simulink model "dronemodel"  (R2023a)
settings: Solver=VariableStepAuto  StartTime=0.0  StopTime=300  RelTol=1e-3
values from neighbouring files (symbols this model uses):
  Ax = 1    [dronevalues.m]
  Ay = 1    [dronevalues.m]
  Az = 1    [dronevalues.m]
  b = 3.59*10^-5    (= 3.59e-05)    [dronevalues.m]
  d = 0.1    [dronevalues.m]
  g = 9.81    [dronevalues.m]
  h = 5    [dronevalues.m]
  Ixx = 0.00963    [dronevalues.m]
  Iyy = 0.00963    [dronevalues.m]
  Izz = 0.019    [dronevalues.m]
  Jr = 0.04439    [dronevalues.m]
  l = 0.24    [dronevalues.m]
  m = 0.9928    [dronevalues.m]
undefined symbols (not defined in the file or in its folder): JSBSim, Rascal110
libraries: SignalEditorBlockLib x9, simulink_extras x7, slpidlib x4, aerolibfltsims x2
settings Model: Creator=ASUS  LastModifiedBy=ASUS

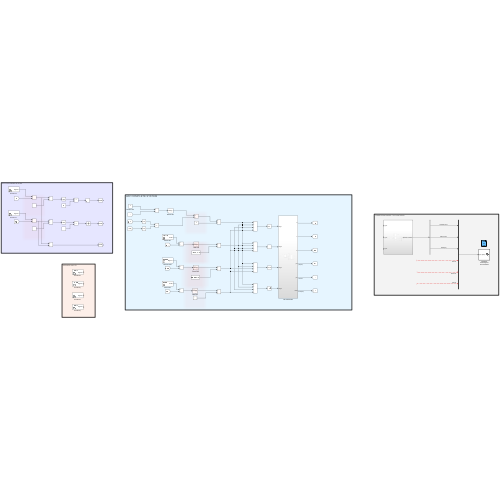
[thumbnail: Simulink's stored preview of the top-level diagram]
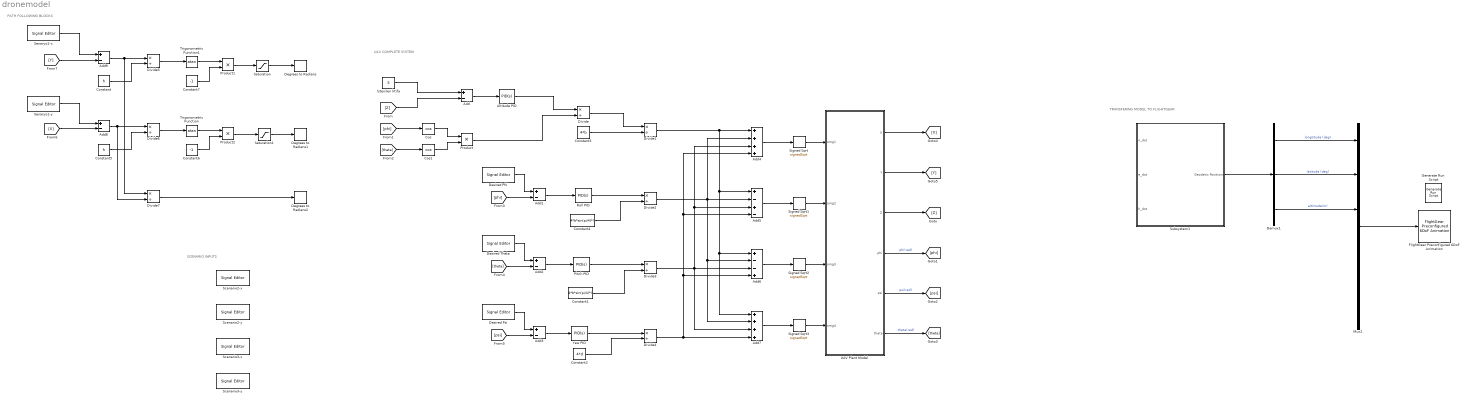
== system dronemodel ==
  note: UAV COMPLETE SYSTEM
  note: TRANSFERING MODEL TO FLIGHTGEAR
  note: PATH FOLLOWING BLOCKS
  note: SCENARIO INPUTS
  Add{,1..3,8..9} (6 alike) : Sum  Inputs=+-
  Add4 : Sum  Inputs=++++
  Add5 : Sum  Inputs=+-+-
  Add6 : Sum  Inputs=+--+
  Add7 : Sum  Inputs=++++
  Altitude PID : slpidlib/PID Controller  Controller=PID  Form=Parallel  TimeDomain=Continuous-time  UseExternalTs=off  SampleTime=-1  IntegratorMethod=Forward Euler  FilterMethod=Forward Euler  ControllerParametersSource=internal  P=1  I=1  UseKiTs=off  D=0  N=100  UseFilter=on  TunerSelectOption=Transfer Function Based (PID Tuner App)  InitialConditionSource=internal  InitialConditionForIntegrator=0  InitialConditionForFilter=0  DifferentiatorICPrevScaledInput=0  ExternalReset=none  TrackingMode=off  Kt=1  LimitOutput=off  SatLimitsSource=internal  UpperSaturationLimit=inf  LowerSaturationLimit=-inf  LinearizeAsGain=on  AntiWindupMode=none  Kb=1  LimitIntegrator=off  UpperIntegratorSaturationLimit=inf  LowerIntegratorSaturationLimit=-inf  POutMin=[]  POutMax=[]  IOutMin=[]  IOutMax=[]  DOutMin=[]  DOutMax=[]  NOutMin=[]  NOutMax=[]  SumOutMin=[]  SumOutMax=[]  SaturationOutMin=[]  SaturationOutMax=[]  PParamMin=[]  PParamMax=[]  IParamMin=[]  IParamMax=[]  DParamMin=[]  DParamMax=[]  NParamMin=[]  NParamMax=[]  KbParamMin=[]  KbParamMax=[]  KtParamMin=[]  KtParamMax=[]  KbOutMin=[]  KbOutMax=[]  KtOutMin=[]  KtOutMax=[]  IntegratorOutMin=[]  IntegratorOutMax=[]  FilterOutMin=[]  FilterOutMax=[]  SumI1OutMin=[]  SumI1OutMax=[]  SumI2OutMin=[]  SumI2OutMax=[]  SumI3OutMin=[]  SumI3OutMax=[]  SumI4OutMin=[]  SumI4OutMax=[]  SumDOutMin=[]  SumDOutMax=[]  DifferentiatorOutMin=[]  DifferentiatorOutMax=[]  FilterDiffOutCoefMin=[]  FilterDiffOutCoefMax=[]  ReciprocalOutMin=[]  ReciprocalOutMax=[]  SumDenOutMin=[]  SumDenOutMax=[]  SumNumOutMin=[]  SumNumOutMax=[]  DivideOutMin=[]  DivideOutMax=[]  UdiffTsProdOutMin=[]  UdiffTsProdOutMax=[]  NTsProdOutMin=[]  NTsProdOutMax=[]  UintegralTsProdOutMin=[]  UintegralTsProdOutMax=[]  UngainTsProdOutMin=[]  UngainTsProdOutMax=[]  ClampingZeroOutDataTypeStr=Inherit: Inherit via back propagation  ClampingZeroOutMin=[]  ClampingZeroOutMax=[]  FilterDenConstantOutDataTypeStr=Inherit: Inherit via back propagation  FilterDenConstantOutMin=[]  FilterDenConstantOutMax=[]  PCopyOutDataTypeStr=Inherit: Inherit via back propagation  PCopyOutMin=[]  PCopyOutMax=[]  NCopyOutDataTypeStr=Inherit: Inherit via back propagation  NCopyOutMin=[]  NCopyOutMax=[]  IntegratorContinuousStateAttributes=''  IntegratorStateMustResolveToSignalObject=off  IntegratorRTWStateStorageClass=Auto  FilterContinuousStateAttributes=''  FilterStateMustResolveToSignalObject=off  FilterRTWStateStorageClass=Auto  ParallelPVariant=InternalParameters  IdealPVariant=Disabled  IVariant=InternalParameters  DVariant=InternalParameters  IntegratorVariant=Continuous  SatVariant=Disabled  AWVariant=Passthrough  PCopyVariant=Disabled  TRVariant=Disabled  FdbkBlocksVariant=Forward  IdealPFdbkVariant=Disabled  SatFdbkVariant=Disabled  DerivativeFilterVariant=ContFilter  NVariant=InternalParameters  NCopyVariant=Disabled  FilterICVariant=InternalICsFilter  IntegratorICVariant=InternalICs  ExternalResetVariant=Disabled  TRSumVariant=Passthrough  SumFdbkVariant=Disabled  SumVariant=Sum_PID  TsampFilterVariant=InternalTs  TsampNgainVariant=Passthrough  TsampIntegralVariant=Disabled_SignalSpec  ExternalSaturationOutDataTypeStr=Inherit: Same as second input
  Constant : Constant  Value=h
  Constant1 : Constant  Value=4*b*sin(pi/4)*l
  Constant2 : Constant  Value=4*d
  Constant3 : Constant  Value=4*b
  Constant4 : Constant  Value=4*b*sin(pi/4)*l
  Constant5 : Constant  Value=h
  Constant6 : Constant  Value=-1
  Constant7 : Constant  Value=-1
  Cos : Trigonometry  Operator=cos
  Cos1 : Trigonometry  Operator=cos
  Degrees to Radians : simulink_extras/Transformations/Degrees to Radians
  Degrees to Radians1 : simulink_extras/Transformations/Degrees to Radians
  Degrees to Radians2 : simulink_extras/Transformations/Degrees to Radians
  Demux1 : Demux  Outputs=3
  Desired Phi : SignalEditorBlockLib/Signal Editor  FileName=phisignal.mat  ActiveScenario=Scenario  ActiveSignal=Pulse  IsBus=off  OutputBusObjectStr=Bus: BusObject  SampleTime=0  Interpolate=off  ZeroCross=off  OutputAfterFinalValue=Setting to zero  Unit=inherit  PreserveSignalName=on  ApplySigPropsToAllScenarios=on
  Desired Psi : SignalEditorBlockLib/Signal Editor  FileName=psisignal.mat  ActiveScenario=Scenario  ActiveSignal=Pulse  IsBus=off  OutputBusObjectStr=Bus: BusObject  SampleTime=0  Interpolate=off  ZeroCross=off  OutputAfterFinalValue=Setting to zero  Unit=inherit  PreserveSignalName=on  ApplySigPropsToAllScenarios=on
  Desired Theta : SignalEditorBlockLib/Signal Editor  FileName=untitled.mat  ActiveScenario=Scenario  ActiveSignal=Signal 1  IsBus=off  OutputBusObjectStr=Bus: BusObject  SampleTime=0  Interpolate=off  ZeroCross=off  OutputAfterFinalValue=Setting to zero  Unit=inherit  PreserveSignalName=on  ApplySigPropsToAllScenarios=on
  Divide{,1..7} (8 alike) : Product  Inputs=*/  RndMeth=Zero  SaturateOnIntegerOverflow=on
  FlightGear Preconfigured 6DoF Animation : aerolibfltsims/FlightGear Preconfigured 6DoF Animation  xFlightGearVersion=v2019.1  DestinationIpAddress=127.0.0.1  DestinationPort=5502  SampleTime=1/100  packetVersion=24
  Generate Run Script : aerolibfltsims/Generate Run Script  Architecture=Win64  dataFlow=Send  GeometryModelName=Rascal110-JSBSim  AirportId=LTAE  RunwayId=21  InitialAltitude=6000  InitialHeading=32  OffsetDistance=0  OffsetAzimuth=0  InstallScenery=on  DisableShaders=off  OriginAddress=127.0.0.1  DestinationPort=5502  OriginPort=5505  LocalAddress=127.0.0.1  OutputFileName=runfg.bat  FlightGearBaseDirectory=C:\FlightGear
  Mux2 : Mux  Inputs=6
  Pitch PID : slpidlib/PID Controller  Controller=PID  Form=Parallel  TimeDomain=Continuous-time  UseExternalTs=off  SampleTime=-1  IntegratorMethod=Forward Euler  FilterMethod=Forward Euler  ControllerParametersSource=internal  P=1  I=1  UseKiTs=off  D=0  N=100  UseFilter=on  TunerSelectOption=Transfer Function Based (PID Tuner App)  InitialConditionSource=internal  InitialConditionForIntegrator=0  InitialConditionForFilter=0  DifferentiatorICPrevScaledInput=0  ExternalReset=none  TrackingMode=off  Kt=1  LimitOutput=off  SatLimitsSource=internal  UpperSaturationLimit=inf  LowerSaturationLimit=-inf  LinearizeAsGain=on  AntiWindupMode=none  Kb=1  LimitIntegrator=off  UpperIntegratorSaturationLimit=inf  LowerIntegratorSaturationLimit=-inf  POutMin=[]  POutMax=[]  IOutMin=[]  IOutMax=[]  DOutMin=[]  DOutMax=[]  NOutMin=[]  NOutMax=[]  SumOutMin=[]  SumOutMax=[]  SaturationOutMin=[]  SaturationOutMax=[]  PParamMin=[]  PParamMax=[]  IParamMin=[]  IParamMax=[]  DParamMin=[]  DParamMax=[]  NParamMin=[]  NParamMax=[]  KbParamMin=[]  KbParamMax=[]  KtParamMin=[]  KtParamMax=[]  KbOutMin=[]  KbOutMax=[]  KtOutMin=[]  KtOutMax=[]  IntegratorOutMin=[]  IntegratorOutMax=[]  FilterOutMin=[]  FilterOutMax=[]  SumI1OutMin=[]  SumI1OutMax=[]  SumI2OutMin=[]  SumI2OutMax=[]  SumI3OutMin=[]  SumI3OutMax=[]  SumI4OutMin=[]  SumI4OutMax=[]  SumDOutMin=[]  SumDOutMax=[]  DifferentiatorOutMin=[]  DifferentiatorOutMax=[]  FilterDiffOutCoefMin=[]  FilterDiffOutCoefMax=[]  ReciprocalOutMin=[]  ReciprocalOutMax=[]  SumDenOutMin=[]  SumDenOutMax=[]  SumNumOutMin=[]  SumNumOutMax=[]  DivideOutMin=[]  DivideOutMax=[]  UdiffTsProdOutMin=[]  UdiffTsProdOutMax=[]  NTsProdOutMin=[]  NTsProdOutMax=[]  UintegralTsProdOutMin=[]  UintegralTsProdOutMax=[]  UngainTsProdOutMin=[]  UngainTsProdOutMax=[]  ClampingZeroOutDataTypeStr=Inherit: Inherit via back propagation  ClampingZeroOutMin=[]  ClampingZeroOutMax=[]  FilterDenConstantOutDataTypeStr=Inherit: Inherit via back propagation  FilterDenConstantOutMin=[]  FilterDenConstantOutMax=[]  PCopyOutDataTypeStr=Inherit: Inherit via back propagation  PCopyOutMin=[]  PCopyOutMax=[]  NCopyOutDataTypeStr=Inherit: Inherit via back propagation  NCopyOutMin=[]  NCopyOutMax=[]  IntegratorContinuousStateAttributes=''  IntegratorStateMustResolveToSignalObject=off  IntegratorRTWStateStorageClass=Auto  FilterContinuousStateAttributes=''  FilterStateMustResolveToSignalObject=off  FilterRTWStateStorageClass=Auto  ParallelPVariant=InternalParameters  IdealPVariant=Disabled  IVariant=InternalParameters  DVariant=InternalParameters  IntegratorVariant=Continuous  SatVariant=Disabled  AWVariant=Passthrough  PCopyVariant=Disabled  TRVariant=Disabled  FdbkBlocksVariant=Forward  IdealPFdbkVariant=Disabled  SatFdbkVariant=Disabled  DerivativeFilterVariant=ContFilter  NVariant=InternalParameters  NCopyVariant=Disabled  FilterICVariant=InternalICsFilter  IntegratorICVariant=InternalICs  ExternalResetVariant=Disabled  TRSumVariant=Passthrough  SumFdbkVariant=Disabled  SumVariant=Sum_PID  TsampFilterVariant=InternalTs  TsampNgainVariant=Passthrough  TsampIntegralVariant=Disabled_SignalSpec  ExternalSaturationOutDataTypeStr=Inherit: Same as second input
  Product : Product
  Product1 : Product
  Product2 : Product
  Roll PID : slpidlib/PID Controller  Controller=PID  Form=Parallel  TimeDomain=Continuous-time  UseExternalTs=off  SampleTime=-1  IntegratorMethod=Forward Euler  FilterMethod=Forward Euler  ControllerParametersSource=internal  P=1  I=1  UseKiTs=off  D=0  N=100  UseFilter=on  TunerSelectOption=Transfer Function Based (PID Tuner App)  InitialConditionSource=internal  InitialConditionForIntegrator=0  InitialConditionForFilter=0  DifferentiatorICPrevScaledInput=0  ExternalReset=none  TrackingMode=off  Kt=1  LimitOutput=off  SatLimitsSource=internal  UpperSaturationLimit=inf  LowerSaturationLimit=-inf  LinearizeAsGain=on  AntiWindupMode=none  Kb=1  LimitIntegrator=off  UpperIntegratorSaturationLimit=inf  LowerIntegratorSaturationLimit=-inf  POutMin=[]  POutMax=[]  IOutMin=[]  IOutMax=[]  DOutMin=[]  DOutMax=[]  NOutMin=[]  NOutMax=[]  SumOutMin=[]  SumOutMax=[]  SaturationOutMin=[]  SaturationOutMax=[]  PParamMin=[]  PParamMax=[]  IParamMin=[]  IParamMax=[]  DParamMin=[]  DParamMax=[]  NParamMin=[]  NParamMax=[]  KbParamMin=[]  KbParamMax=[]  KtParamMin=[]  KtParamMax=[]  KbOutMin=[]  KbOutMax=[]  KtOutMin=[]  KtOutMax=[]  IntegratorOutMin=[]  IntegratorOutMax=[]  FilterOutMin=[]  FilterOutMax=[]  SumI1OutMin=[]  SumI1OutMax=[]  SumI2OutMin=[]  SumI2OutMax=[]  SumI3OutMin=[]  SumI3OutMax=[]  SumI4OutMin=[]  SumI4OutMax=[]  SumDOutMin=[]  SumDOutMax=[]  DifferentiatorOutMin=[]  DifferentiatorOutMax=[]  FilterDiffOutCoefMin=[]  FilterDiffOutCoefMax=[]  ReciprocalOutMin=[]  ReciprocalOutMax=[]  SumDenOutMin=[]  SumDenOutMax=[]  SumNumOutMin=[]  SumNumOutMax=[]  DivideOutMin=[]  DivideOutMax=[]  UdiffTsProdOutMin=[]  UdiffTsProdOutMax=[]  NTsProdOutMin=[]  NTsProdOutMax=[]  UintegralTsProdOutMin=[]  UintegralTsProdOutMax=[]  UngainTsProdOutMin=[]  UngainTsProdOutMax=[]  ClampingZeroOutDataTypeStr=Inherit: Inherit via back propagation  ClampingZeroOutMin=[]  ClampingZeroOutMax=[]  FilterDenConstantOutDataTypeStr=Inherit: Inherit via back propagation  FilterDenConstantOutMin=[]  FilterDenConstantOutMax=[]  PCopyOutDataTypeStr=Inherit: Inherit via back propagation  PCopyOutMin=[]  PCopyOutMax=[]  NCopyOutDataTypeStr=Inherit: Inherit via back propagation  NCopyOutMin=[]  NCopyOutMax=[]  IntegratorContinuousStateAttributes=''  IntegratorStateMustResolveToSignalObject=off  IntegratorRTWStateStorageClass=Auto  FilterContinuousStateAttributes=''  FilterStateMustResolveToSignalObject=off  FilterRTWStateStorageClass=Auto  ParallelPVariant=InternalParameters  IdealPVariant=Disabled  IVariant=InternalParameters  DVariant=InternalParameters  IntegratorVariant=Continuous  SatVariant=Disabled  AWVariant=Passthrough  PCopyVariant=Disabled  TRVariant=Disabled  FdbkBlocksVariant=Forward  IdealPFdbkVariant=Disabled  SatFdbkVariant=Disabled  DerivativeFilterVariant=ContFilter  NVariant=InternalParameters  NCopyVariant=Disabled  FilterICVariant=InternalICsFilter  IntegratorICVariant=InternalICs  ExternalResetVariant=Disabled  TRSumVariant=Passthrough  SumFdbkVariant=Disabled  SumVariant=Sum_PID  TsampFilterVariant=InternalTs  TsampNgainVariant=Passthrough  TsampIntegralVariant=Disabled_SignalSpec  ExternalSaturationOutDataTypeStr=Inherit: Same as second input
  Saturation : Saturate  UpperLimit=20  LowerLimit=-20
  Saturation1 : Saturate  UpperLimit=20  LowerLimit=-20
  Scenario2-x : SignalEditorBlockLib/Signal Editor  FileName=Senaryo2X.mat  ActiveScenario=Scenario  ActiveSignal=Signal 1  IsBus=off  OutputBusObjectStr=Bus: BusObject  SampleTime=0  Interpolate=off  ZeroCross=off  OutputAfterFinalValue=Setting to zero  Unit=inherit  PreserveSignalName=on  ApplySigPropsToAllScenarios=on
  Scenario2-y : SignalEditorBlockLib/Signal Editor  FileName=C:\Users\s22734\Desktop\Senaryo2Y.mat  ActiveScenario=Scenario  ActiveSignal=Signal 1  IsBus=off  OutputBusObjectStr=Bus: BusObject  SampleTime=0  Interpolate=off  ZeroCross=off  OutputAfterFinalValue=Setting to zero  Unit=inherit  PreserveSignalName=on  ApplySigPropsToAllScenarios=on
  Scenario3-x : SignalEditorBlockLib/Signal Editor  FileName=Senaryo3X.mat  ActiveScenario=Scenario  ActiveSignal=Signal 1  IsBus=off  OutputBusObjectStr=Bus: BusObject  SampleTime=0  Interpolate=off  ZeroCross=off  OutputAfterFinalValue=Setting to zero  Unit=inherit  PreserveSignalName=on  ApplySigPropsToAllScenarios=on
  Scenario3-y : SignalEditorBlockLib/Signal Editor  FileName=Senaryo3Y.mat  ActiveScenario=Scenario  ActiveSignal=Signal 1  IsBus=off  OutputBusObjectStr=Bus: BusObject  SampleTime=0  Interpolate=off  ZeroCross=off  OutputAfterFinalValue=Setting to zero  Unit=inherit  PreserveSignalName=on  ApplySigPropsToAllScenarios=on
  Senaryo1-x : SignalEditorBlockLib/Signal Editor  FileName=C:\Users\s22734\Desktop\Senaryo1X.mat  ActiveScenario=Scenario  ActiveSignal=Signal 1  IsBus=off  OutputBusObjectStr=Bus: BusObject  SampleTime=0  Interpolate=off  ZeroCross=off  OutputAfterFinalValue=Setting to zero  Unit=inherit  PreserveSignalName=on  ApplySigPropsToAllScenarios=on
  Senaryo1-y : SignalEditorBlockLib/Signal Editor  FileName=C:\Users\s22734\Desktop\Senaryo1Y.mat  ActiveScenario=Scenario  ActiveSignal=Signal 1  IsBus=off  OutputBusObjectStr=Bus: BusObject  SampleTime=0  Interpolate=off  ZeroCross=off  OutputAfterFinalValue=Setting to zero  Unit=inherit  PreserveSignalName=on  ApplySigPropsToAllScenarios=on
  Signed Sqrt{,1..3} (4 alike) : Sqrt  Operator=signedSqrt
  Subsystem1 : Subsystem
  Trigonometric Function : Trigonometry  Operator=atan
  Trigonometric Function1 : Trigonometry  Operator=atan
  UAV Plant Model : Subsystem
  Yaw PID : slpidlib/PID Controller  Controller=PID  Form=Parallel  TimeDomain=Continuous-time  UseExternalTs=off  SampleTime=-1  IntegratorMethod=Forward Euler  FilterMethod=Forward Euler  ControllerParametersSource=internal  P=1  I=1  UseKiTs=off  D=0  N=100  UseFilter=on  TunerSelectOption=Transfer Function Based (PID Tuner App)  InitialConditionSource=internal  InitialConditionForIntegrator=0  InitialConditionForFilter=0  DifferentiatorICPrevScaledInput=0  ExternalReset=none  TrackingMode=off  Kt=1  LimitOutput=off  SatLimitsSource=internal  UpperSaturationLimit=inf  LowerSaturationLimit=-inf  LinearizeAsGain=on  AntiWindupMode=none  Kb=1  LimitIntegrator=off  UpperIntegratorSaturationLimit=inf  LowerIntegratorSaturationLimit=-inf  POutMin=[]  POutMax=[]  IOutMin=[]  IOutMax=[]  DOutMin=[]  DOutMax=[]  NOutMin=[]  NOutMax=[]  SumOutMin=[]  SumOutMax=[]  SaturationOutMin=[]  SaturationOutMax=[]  PParamMin=[]  PParamMax=[]  IParamMin=[]  IParamMax=[]  DParamMin=[]  DParamMax=[]  NParamMin=[]  NParamMax=[]  KbParamMin=[]  KbParamMax=[]  KtParamMin=[]  KtParamMax=[]  KbOutMin=[]  KbOutMax=[]  KtOutMin=[]  KtOutMax=[]  IntegratorOutMin=[]  IntegratorOutMax=[]  FilterOutMin=[]  FilterOutMax=[]  SumI1OutMin=[]  SumI1OutMax=[]  SumI2OutMin=[]  SumI2OutMax=[]  SumI3OutMin=[]  SumI3OutMax=[]  SumI4OutMin=[]  SumI4OutMax=[]  SumDOutMin=[]  SumDOutMax=[]  DifferentiatorOutMin=[]  DifferentiatorOutMax=[]  FilterDiffOutCoefMin=[]  FilterDiffOutCoefMax=[]  ReciprocalOutMin=[]  ReciprocalOutMax=[]  SumDenOutMin=[]  SumDenOutMax=[]  SumNumOutMin=[]  SumNumOutMax=[]  DivideOutMin=[]  DivideOutMax=[]  UdiffTsProdOutMin=[]  UdiffTsProdOutMax=[]  NTsProdOutMin=[]  NTsProdOutMax=[]  UintegralTsProdOutMin=[]  UintegralTsProdOutMax=[]  UngainTsProdOutMin=[]  UngainTsProdOutMax=[]  ClampingZeroOutDataTypeStr=Inherit: Inherit via back propagation  ClampingZeroOutMin=[]  ClampingZeroOutMax=[]  FilterDenConstantOutDataTypeStr=Inherit: Inherit via back propagation  FilterDenConstantOutMin=[]  FilterDenConstantOutMax=[]  PCopyOutDataTypeStr=Inherit: Inherit via back propagation  PCopyOutMin=[]  PCopyOutMax=[]  NCopyOutDataTypeStr=Inherit: Inherit via back propagation  NCopyOutMin=[]  NCopyOutMax=[]  IntegratorContinuousStateAttributes=''  IntegratorStateMustResolveToSignalObject=off  IntegratorRTWStateStorageClass=Auto  FilterContinuousStateAttributes=''  FilterStateMustResolveToSignalObject=off  FilterRTWStateStorageClass=Auto  ParallelPVariant=InternalParameters  IdealPVariant=Disabled  IVariant=InternalParameters  DVariant=InternalParameters  IntegratorVariant=Continuous  SatVariant=Disabled  AWVariant=Passthrough  PCopyVariant=Disabled  TRVariant=Disabled  FdbkBlocksVariant=Forward  IdealPFdbkVariant=Disabled  SatFdbkVariant=Disabled  DerivativeFilterVariant=ContFilter  NVariant=InternalParameters  NCopyVariant=Disabled  FilterICVariant=InternalICsFilter  IntegratorICVariant=InternalICs  ExternalResetVariant=Disabled  TRSumVariant=Passthrough  SumFdbkVariant=Disabled  SumVariant=Sum_PID  TsampFilterVariant=InternalTs  TsampNgainVariant=Passthrough  TsampIntegralVariant=Disabled_SignalSpec  ExternalSaturationOutDataTypeStr=Inherit: Same as second input
  İstenilen İrtifa : Constant  Value=5
  wires:
  Add4/1 -> Signed Sqrt/1
  Add5/1 -> Signed Sqrt1/1
  Add6/1 -> Signed Sqrt2/1
  Add7/1 -> Signed Sqrt3/1
  UAV Plant Model/1(X) -> [X]
  UAV Plant Model/2(Y) -> [Y]
  İstenilen İrtifa/1 -> Add/1
  Add/1 -> Altitude PID/1
  UAV Plant Model/3(Z) -> [Z]
  [Z] -> Add/2
  [phi] -> Cos/1
  [theta] -> Cos1/1
  Cos/1 -> Product/1
  Cos1/1 -> Product/2
  Product/1 -> Divide/2
  Altitude PID/1 -> Divide/1
  [phi] -> Add1/2
  Add1/1 -> Roll PID/1
  [theta] -> Add2/2
  Add2/1 -> Pitch PID/1
  [psi] -> Add3/2
  Add3/1 -> Yaw PID/1
  Divide/1 -> Divide1/1
  Constant3/1 -> Divide1/2
  Roll PID/1 -> Divide2/1
  Constant4/1 -> Divide2/2
  Pitch PID/1 -> Divide3/1
  Constant1/1 -> Divide3/2
  Yaw PID/1 -> Divide4/1
  Constant2/1 -> Divide4/2
  Divide1/1 -> Add6/1, Add7/1, Add5/1, Add4/1
  Divide2/1 -> Add7/2, Add6/2, Add5/2, Add4/2
  Divide4/1 -> Add4/4, Add5/4, Add6/4, Add7/4
  Divide3/1 -> Add7/3, Add6/3, Add4/3, Add5/3
  Signed Sqrt/1 -> UAV Plant Model/1(omg1)
  Signed Sqrt1/1 -> UAV Plant Model/2(omg2)
  Signed Sqrt2/1 -> UAV Plant Model/3(omg3)
  Signed Sqrt3/1 -> UAV Plant Model/4(omg4)
  ? -> Mux2/5  "theta(rad)"
  Demux1/2 -> Mux2/2  "latitude (deg)"
  Demux1/1 -> Mux2/1  "longtitude (deg)"
  Mux2/1 -> FlightGear Preconfigured 6DoF Animation/1
  ? -> Mux2/6  "psi(rad)"
  ? -> Mux2/4  "phi(rad)"
  Demux1/3 -> Mux2/3  "altittude(m)"
  Subsystem1/1(Geodetic Positions) -> Demux1/1
  [X] -> Add8/2
  [Y] -> Add9/2
  Add9/1 -> Divide5/1, Divide7/1
  Add8/1 -> Divide6/1, Divide7/2
  Constant/1 -> Divide5/2
  Constant5/1 -> Divide6/2
  Divide5/1 -> Trigonometric Function1/1
  Divide6/1 -> Trigonometric Function/1
  Trigonometric Function1/1 -> Product1/1
  Trigonometric Function/1 -> Product2/1
  Senaryo1-x/1 -> Add9/1
  Senaryo1-y/1 -> Add8/1
  Product1/1 -> Saturation/1
  Product2/1 -> Saturation1/1
  Constant7/1 -> Product1/2
  Constant6/1 -> Product2/2
  Saturation/1 -> Degrees to Radians/1
  Saturation1/1 -> Degrees to Radians1/1
  Divide7/1 -> Degrees to Radians2/1
  UAV Plant Model/4(phi) -> [phi]  "phi(rad)"
  UAV Plant Model/5(psi) -> [psi]  "psi(rad)"
  UAV Plant Model/6(theta) -> [theta]  "theta(rad)"
  Desired Phi/1 -> Add1/1
  Desired Theta/1 -> Add2/1
  Desired Psi/1 -> Add3/1

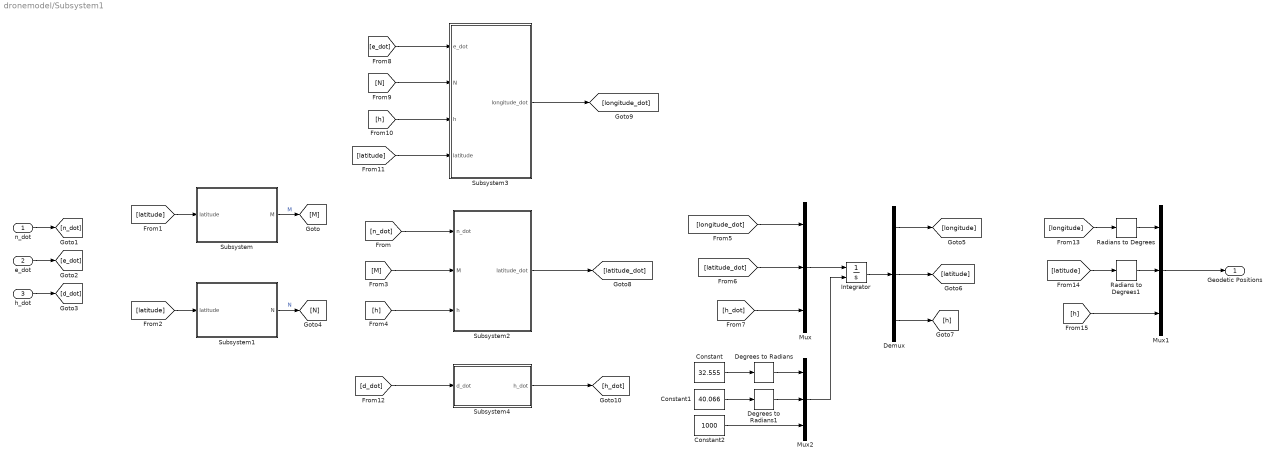
== system dronemodel/Subsystem1 ==
  n_dot : Inport
  e_dot : Inport  Port=2
  h_dot : Inport  Port=3
  Constant : Constant  Value=32.555
  Constant1 : Constant  Value=40.066
  Constant2 : Constant  Value=1000
  Degrees to Radians : simulink_extras/Transformations/Degrees to Radians
  Degrees to Radians1 : simulink_extras/Transformations/Degrees to Radians
  Demux : Demux  Outputs=3
  Integrator : Integrator  InitialConditionSource=external  InitialCondition=[32.555;40.066;3000]
  Mux : Mux  Inputs=3
  Mux1 : Mux  Inputs=3
  Mux2 : Mux  Inputs=3
  Radians to Degrees : simulink_extras/Transformations/Radians to Degrees
  Radians to Degrees1 : simulink_extras/Transformations/Radians to Degrees
  Subsystem : Subsystem
  Subsystem1 : Subsystem
  Subsystem2 : Subsystem
  Subsystem3 : Subsystem
  Subsystem4 : Subsystem
  Geodetic Positions : Outport
  wires:
  e_dot/1 -> [e_dot]
  n_dot/1 -> [n_dot]
  h_dot/1 -> [d_dot]
  [latitude] -> Subsystem/1(latitude)
  Subsystem/1(M) -> [M]  "M"
  [latitude] -> Subsystem1/1(latitude)
  Subsystem1/1(N) -> [N]  "N"
  [longitude_dot] -> Mux/1
  [latitude_dot] -> Mux/2
  [h_dot] -> Mux/3
  Mux/1 -> Integrator/1
  Integrator/1 -> Demux/1
  Demux/1 -> [longitude]
  Demux/3 -> [h]
  Demux/2 -> [latitude]
  [n_dot] -> Subsystem2/1(n_dot)
  [M] -> Subsystem2/2(M)
  [h] -> Subsystem2/3(h)
  Subsystem2/1(latitude_dot) -> [latitude_dot]
  [e_dot] -> Subsystem3/1(e_dot)
  [N] -> Subsystem3/2(N)
  [h] -> Subsystem3/3(h)
  [latitude] -> Subsystem3/4(latitude)
  Subsystem3/1(longitude_dot) -> [longitude_dot]
  [d_dot] -> Subsystem4/1(d_dot)
  Subsystem4/1(h_dot) -> [h_dot]
  Mux1/1 -> Geodetic Positions/1
  [longitude] -> Radians to Degrees/1
  [latitude] -> Radians to Degrees1/1
  [h] -> Mux1/3
  Radians to Degrees1/1 -> Mux1/2
  Radians to Degrees/1 -> Mux1/1
  Constant/1 -> Degrees to Radians/1
  Degrees to Radians/1 -> Mux2/1
  Constant1/1 -> Degrees to Radians1/1
  Degrees to Radians1/1 -> Mux2/2
  Constant2/1 -> Mux2/3
  Mux2/1 -> Integrator/2

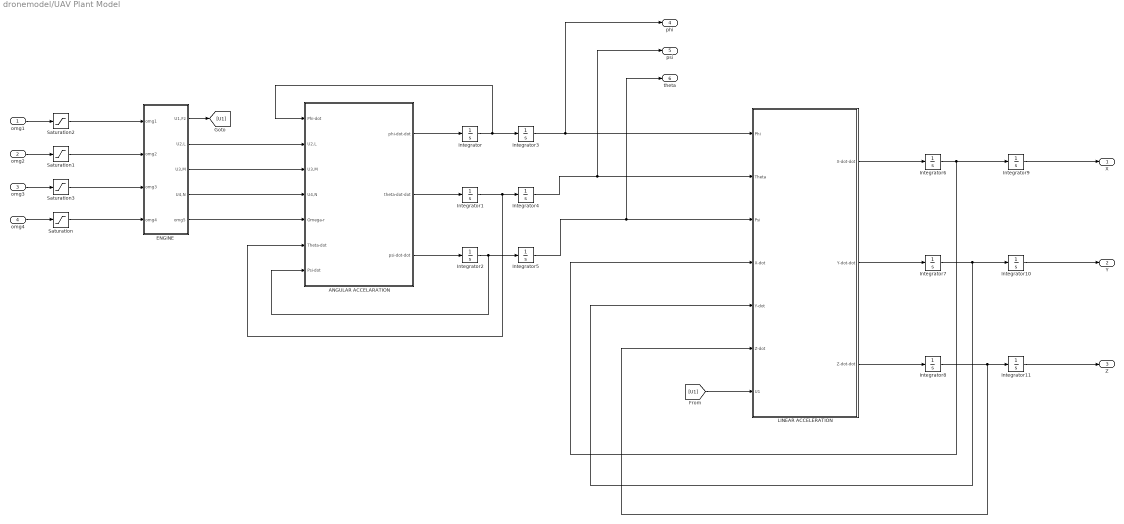
== system dronemodel/UAV Plant Model ==
  omg1 : Inport
  omg2 : Inport  Port=2
  omg3 : Inport  Port=3
  omg4 : Inport  Port=4
  ANGULAR ACCELARATION : Subsystem
  ENGINE : Subsystem
  Integrator{,1..2,6..10} (8 alike) : Integrator
  Integrator11 : Integrator  LimitOutput=on  LowerSaturationLimit=0
  Integrator3 : Integrator  WrapState=on
  Integrator4 : Integrator  WrapState=on
  Integrator5 : Integrator  WrapState=on
  LINEAR ACCELERATION : Subsystem
  Saturation{,1..3} (4 alike) : Saturate
  X : Outport
  Y : Outport  Port=2
  Z : Outport  Port=3
  phi : Outport  Port=4
  psi : Outport  Port=5
  theta : Outport  Port=6
  wires:
  ENGINE/4(U4,N) -> ANGULAR ACCELARATION/4(U4,N)
  Integrator11/1 -> Z/1
  Integrator2/1 -> ANGULAR ACCELARATION/7(Psi-dot), Integrator5/1
  Integrator1/1 -> ANGULAR ACCELARATION/6(Theta-dot), Integrator4/1
  Integrator7/1 -> LINEAR ACCELERATION/5(Y-dot), Integrator10/1
  ENGINE/2(U2,L) -> ANGULAR ACCELARATION/2(U2,L)
  omg1/1 -> Saturation2/1
  Integrator5/1 -> theta/1, LINEAR ACCELERATION/3(Psi)
  LINEAR ACCELERATION/3(Z-dot-dot) -> Integrator8/1
  omg3/1 -> Saturation3/1
  ENGINE/3(U3,M) -> ANGULAR ACCELARATION/3(U3,M)
  omg2/1 -> Saturation1/1
  Integrator/1 -> ANGULAR ACCELARATION/1(Phi-dot), Integrator3/1
  ENGINE/1(U1,Fz) -> [U1]
  Integrator10/1 -> Y/1
  Integrator6/1 -> LINEAR ACCELERATION/4(X-dot), Integrator9/1
  ENGINE/5(omg5) -> ANGULAR ACCELARATION/5(Omega-r)
  [U1] -> LINEAR ACCELERATION/7(U1)
  ANGULAR ACCELARATION/1(phi-dot-dot) -> Integrator/1
  ANGULAR ACCELARATION/3(psi-dot-dot) -> Integrator2/1
  Integrator4/1 -> psi/1, LINEAR ACCELERATION/2(Theta)
  Integrator9/1 -> X/1
  LINEAR ACCELERATION/2(Y-dot-dot) -> Integrator7/1
  Integrator3/1 -> phi/1, LINEAR ACCELERATION/1(Phi)
  omg4/1 -> Saturation/1
  ANGULAR ACCELARATION/2(theta-dot-dot) -> Integrator1/1
  LINEAR ACCELERATION/1(X-dot-dot) -> Integrator6/1
  Integrator8/1 -> LINEAR ACCELERATION/6(Z-dot), Integrator11/1
  Saturation1/1 -> ENGINE/2(omg2)
  Saturation2/1 -> ENGINE/1(omg1)
  Saturation3/1 -> ENGINE/3(omg3)
  Saturation/1 -> ENGINE/4(omg4)

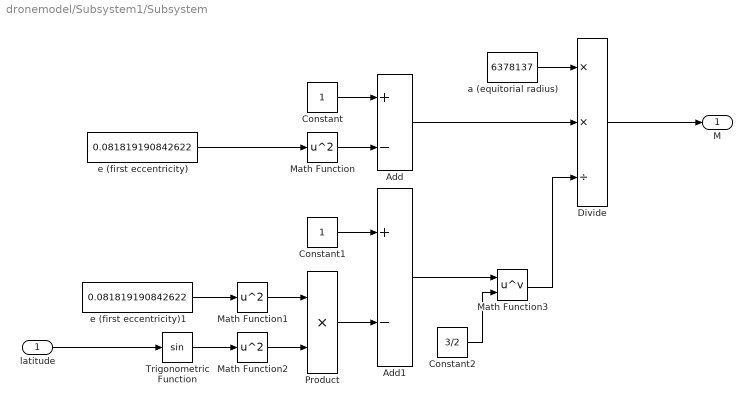
== system dronemodel/Subsystem1/Subsystem ==
  latitude : Inport
  Add : Sum  Inputs=+-
  Add1 : Sum  Inputs=+-
  Constant : Constant
  Constant1 : Constant
  Constant2 : Constant  Value=3/2
  Divide : Product  Inputs=**/
  Math Function : Math  Operator=square
  Math Function1 : Math  Operator=square
  Math Function2 : Math  Operator=square
  Math Function3 : Math  Operator=pow
  Product : Product
  Trigonometric Function : Trigonometry
  a (equitorial radius) : Constant  Value=6378137
  e (first eccentricity) : Constant  Value=0.081819190842622
  e (first eccentricity)1 : Constant  Value=0.081819190842622
  M : Outport
  wires:
  Constant1/1 -> Add1/1
  Add/1 -> Divide/2
  Add1/1 -> Math Function3/1
  Constant2/1 -> Math Function3/2
  Product/1 -> Add1/2
  a (equitorial radius)/1 -> Divide/1
  e (first eccentricity)1/1 -> Math Function1/1
  latitude/1 -> Trigonometric Function/1
  Math Function/1 -> Add/2
  Constant/1 -> Add/1
  Trigonometric Function/1 -> Math Function2/1
  e (first eccentricity)/1 -> Math Function/1
  Math Function1/1 -> Product/1
  Math Function2/1 -> Product/2
  Math Function3/1 -> Divide/3
  Divide/1 -> M/1

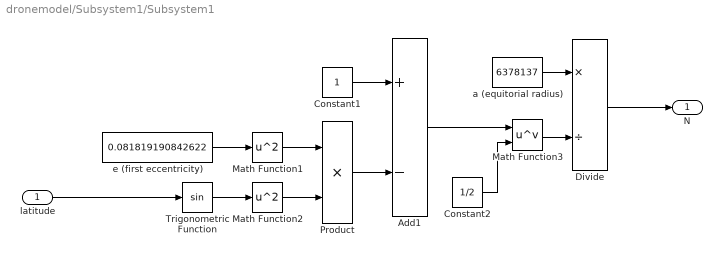
== system dronemodel/Subsystem1/Subsystem1 ==
  latitude : Inport
  Add1 : Sum  Inputs=+-
  Constant1 : Constant
  Constant2 : Constant  Value=1/2
  Divide : Product  Inputs=*/
  Math Function1 : Math  Operator=square
  Math Function2 : Math  Operator=square
  Math Function3 : Math  Operator=pow
  Product : Product
  Trigonometric Function : Trigonometry
  a (equitorial radius) : Constant  Value=6378137
  e (first eccentricity) : Constant  Value=0.081819190842622
  N : Outport
  wires:
  Math Function1/1 -> Product/1
  Product/1 -> Add1/2
  Constant2/1 -> Math Function3/2
  Constant1/1 -> Add1/1
  Add1/1 -> Math Function3/1
  latitude/1 -> Trigonometric Function/1
  Math Function3/1 -> Divide/2
  Math Function2/1 -> Product/2
  Trigonometric Function/1 -> Math Function2/1
  e (first eccentricity)/1 -> Math Function1/1
  a (equitorial radius)/1 -> Divide/1
  Divide/1 -> N/1

== system dronemodel/Subsystem1/Subsystem2 ==
  n_dot : Inport
  M : Inport  Port=2
  h : Inport  Port=3
  Add : Sum
  Divide : Product  Inputs=*/
  latitude_dot : Outport
  wires:
  Add/1 -> Divide/2
  Divide/1 -> latitude_dot/1
  M/1 -> Add/1
  n_dot/1 -> Divide/1
  h/1 -> Add/2

== system dronemodel/Subsystem1/Subsystem3 ==
  e_dot : Inport
  N : Inport  Port=2
  h : Inport  Port=3
  latitude : Inport  Port=4
  Add : Sum
  Divide : Product  Inputs=*//
  Trigonometric Function : Trigonometry  Operator=cos
  longitude_dot : Outport
  wires:
  Trigonometric Function/1 -> Divide/3
  Divide/1 -> longitude_dot/1
  Add/1 -> Divide/2
  latitude/1 -> Trigonometric Function/1
  N/1 -> Add/1
  e_dot/1 -> Divide/1
  h/1 -> Add/2

== system dronemodel/Subsystem1/Subsystem4 ==
  d_dot : Inport
  Gain : Gain  Gain=-1
  h_dot : Outport
  wires:
  Gain/1 -> h_dot/1
  d_dot/1 -> Gain/1

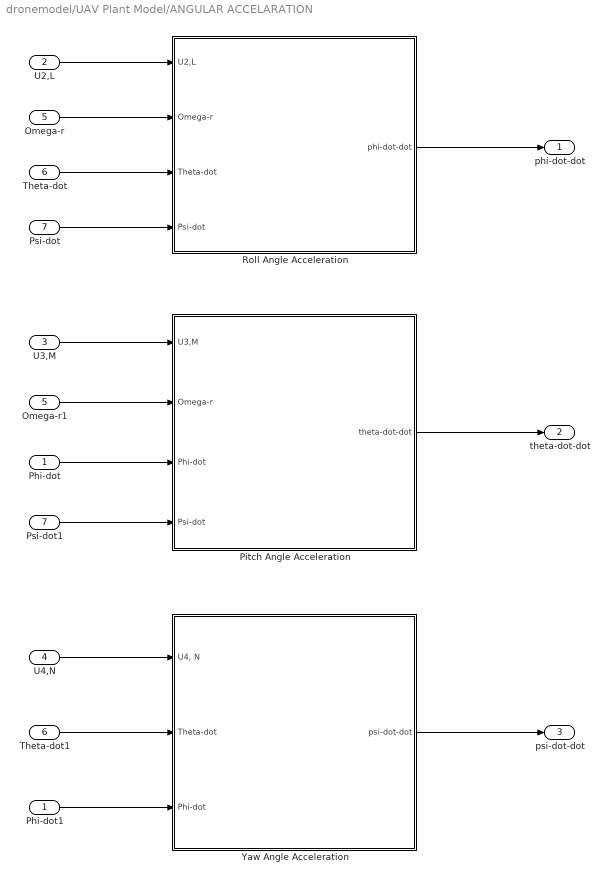
== system dronemodel/UAV Plant Model/ANGULAR ACCELARATION ==
  Phi-dot : Inport
  U2,L : Inport  Port=2
  U3,M : Inport  Port=3
  U4,N : Inport  Port=4
  Omega-r : Inport  Port=5
  Theta-dot : Inport  Port=6
  Psi-dot : Inport  Port=7
  Omega-r1 : InportShadow  Port=5
  Phi-dot1 : InportShadow
  Pitch Angle Acceleration : Subsystem
  Psi-dot1 : InportShadow  Port=7
  Roll Angle Acceleration : Subsystem
  Theta-dot1 : InportShadow  Port=6
  Yaw Angle Acceleration : Subsystem
  phi-dot-dot : Outport
  theta-dot-dot : Outport  Port=2
  psi-dot-dot : Outport  Port=3
  wires:
  U2,L/1 -> Roll Angle Acceleration/1(U2,L)
  Omega-r/1 -> Roll Angle Acceleration/2(Omega-r)
  Theta-dot/1 -> Roll Angle Acceleration/3(Theta-dot)
  Psi-dot/1 -> Roll Angle Acceleration/4(Psi-dot)
  Roll Angle Acceleration/1(phi-dot-dot) -> phi-dot-dot/1
  Pitch Angle Acceleration/1(theta-dot-dot) -> theta-dot-dot/1
  Yaw Angle Acceleration/1(psi-dot-dot) -> psi-dot-dot/1
  U3,M/1 -> Pitch Angle Acceleration/1(U3,M)
  Omega-r1/1 -> Pitch Angle Acceleration/2(Omega-r)
  Phi-dot/1 -> Pitch Angle Acceleration/3(Phi-dot)
  Psi-dot1/1 -> Pitch Angle Acceleration/4(Psi-dot)
  U4,N/1 -> Yaw Angle Acceleration/1("U4, N")
  Theta-dot1/1 -> Yaw Angle Acceleration/2(Theta-dot)
  Phi-dot1/1 -> Yaw Angle Acceleration/3(Phi-dot)

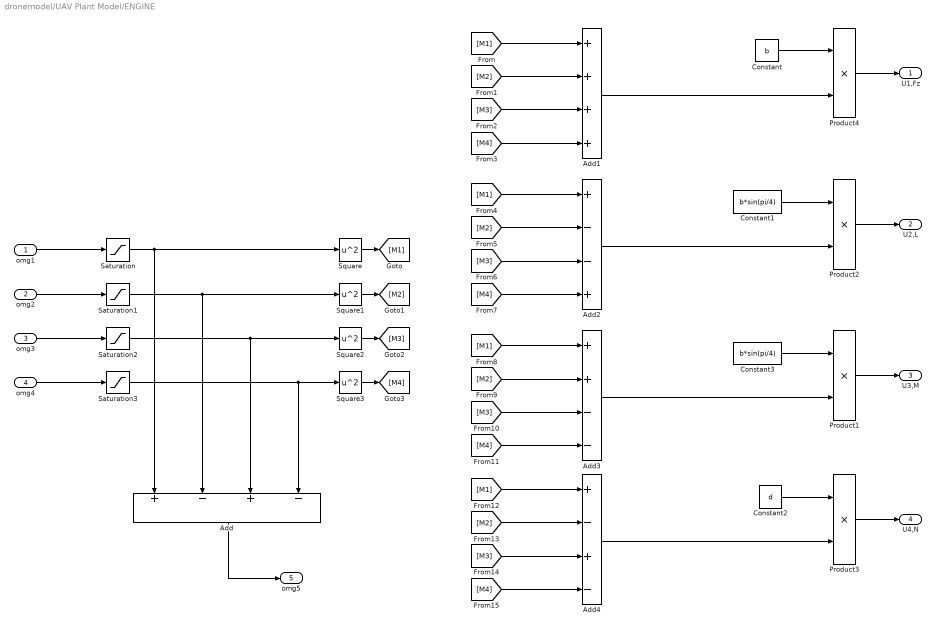
== system dronemodel/UAV Plant Model/ENGINE ==
  omg1 : Inport
  omg2 : Inport  Port=2
  omg3 : Inport  Port=3
  omg4 : Inport  Port=4
  Add : Sum  Inputs=+-+-
  Add1 : Sum  Inputs=++++
  Add2 : Sum  Inputs=+--+
  Add3 : Sum  Inputs=++--
  Add4 : Sum  Inputs=+-+-
  Constant : Constant  Value=b
  Constant1 : Constant  Value=b*sin(pi/4)
  Constant2 : Constant  Value=d
  Constant3 : Constant  Value=b*sin(pi/4)
  Product{1..4} (4 alike) : Product
  Saturation{,1..3} (4 alike) : Saturate
  Square{,1..3} (4 alike) : Math  Operator=square
  U1,Fz : Outport
  U2,L : Outport  Port=2
  U3,M : Outport  Port=3
  U4,N : Outport  Port=4
  omg5 : Outport  Port=5
  wires:
  omg1/1 -> Saturation/1
  omg3/1 -> Saturation2/1
  Saturation/1 -> Add/1, Square/1
  Saturation2/1 -> Add/3, Square2/1
  Saturation3/1 -> Add/4, Square3/1
  omg4/1 -> Saturation3/1
  Square1/1 -> [M2]
  Saturation1/1 -> Add/2, Square1/1
  Square2/1 -> [M3]
  Square/1 -> [M1]
  Square3/1 -> [M4]
  omg2/1 -> Saturation1/1
  Add/1 -> omg5/1
  [M1] -> Add1/1
  [M2] -> Add1/2
  [M3] -> Add1/3
  [M4] -> Add1/4
  [M1] -> Add3/1
  [M2] -> Add3/2
  [M3] -> Add3/3
  [M4] -> Add3/4
  [M1] -> Add4/1
  [M2] -> Add4/2
  [M3] -> Add4/3
  [M4] -> Add4/4
  [M1] -> Add2/1
  [M2] -> Add2/2
  [M3] -> Add2/3
  [M4] -> Add2/4
  Add1/1 -> Product4/2
  Add2/1 -> Product2/2
  Add3/1 -> Product1/2
  Add4/1 -> Product3/2
  Constant2/1 -> Product3/1
  Constant1/1 -> Product2/1
  Constant3/1 -> Product1/1
  Constant/1 -> Product4/1
  Product4/1 -> U1,Fz/1
  Product3/1 -> U4,N/1
  Product1/1 -> U3,M/1
  Product2/1 -> U2,L/1

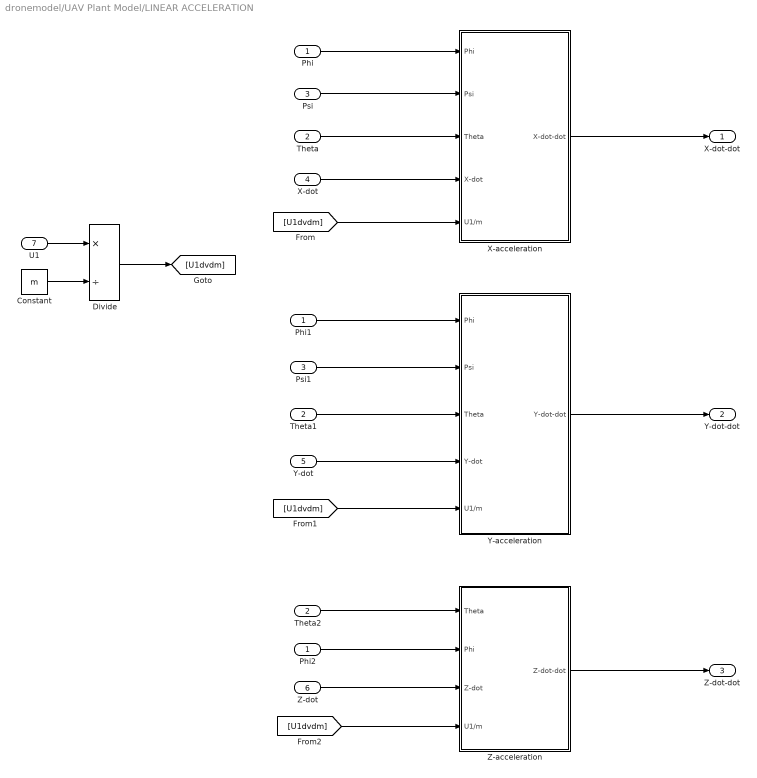
== system dronemodel/UAV Plant Model/LINEAR ACCELERATION ==
  Phi : Inport
  Theta : Inport  Port=2
  Psi : Inport  Port=3
  X-dot : Inport  Port=4
  Y-dot : Inport  Port=5
  Z-dot : Inport  Port=6
  U1 : Inport  Port=7
  Constant : Constant  Value=m
  Divide : Product  Inputs=*/  RndMeth=Zero  SaturateOnIntegerOverflow=on
  Phi1 : InportShadow
  Phi2 : InportShadow
  Psi1 : InportShadow  Port=3
  Theta1 : InportShadow  Port=2
  Theta2 : InportShadow  Port=2
  X-acceleration : Subsystem
  Y-acceleration : Subsystem
  Z-acceleration : Subsystem
  X-dot-dot : Outport
  Y-dot-dot : Outport  Port=2
  Z-dot-dot : Outport  Port=3
  wires:
  Phi/1 -> X-acceleration/1(Phi)
  X-acceleration/1(X-dot-dot) -> X-dot-dot/1
  Y-acceleration/1(Y-dot-dot) -> Y-dot-dot/1
  Z-acceleration/1(Z-dot-dot) -> Z-dot-dot/1
  Psi/1 -> X-acceleration/2(Psi)
  Theta/1 -> X-acceleration/3(Theta)
  X-dot/1 -> X-acceleration/4(X-dot)
  U1/1 -> Divide/1
  Constant/1 -> Divide/2
  Divide/1 -> [U1dvdm]
  [U1dvdm] -> X-acceleration/5(U1/m)
  Phi1/1 -> Y-acceleration/1(Phi)
  Psi1/1 -> Y-acceleration/2(Psi)
  Theta1/1 -> Y-acceleration/3(Theta)
  Y-dot/1 -> Y-acceleration/4(Y-dot)
  [U1dvdm] -> Y-acceleration/5(U1/m)
  Z-dot/1 -> Z-acceleration/3(Z-dot)
  Theta2/1 -> Z-acceleration/1(Theta)
  Phi2/1 -> Z-acceleration/2(Phi)
  [U1dvdm] -> Z-acceleration/4(U1/m)

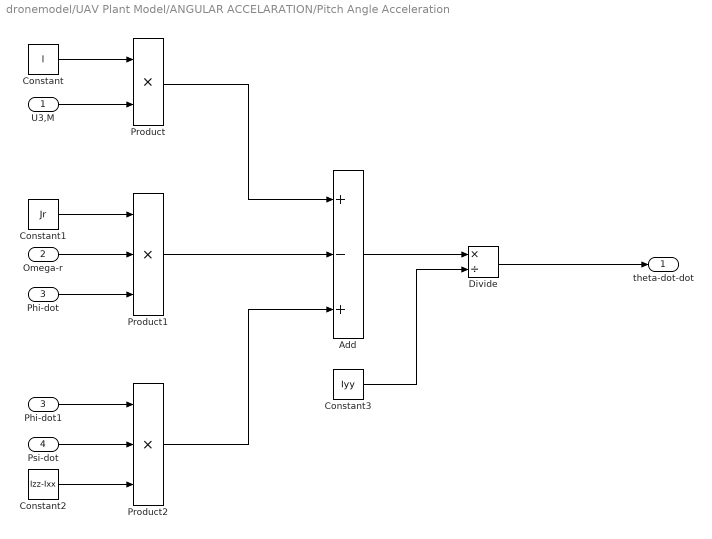
== system dronemodel/UAV Plant Model/ANGULAR ACCELARATION/Pitch Angle Acceleration ==
  U3,M : Inport
  Omega-r : Inport  Port=2
  Phi-dot : Inport  Port=3
  Psi-dot : Inport  Port=4
  Add : Sum  Inputs=+-+
  Constant : Constant  Value=l
  Constant1 : Constant  Value=Jr
  Constant2 : Constant  Value=Izz-Ixx
  Constant3 : Constant  Value=Iyy
  Divide : Product  Inputs=*/
  Phi-dot1 : InportShadow  Port=3
  Product : Product
  Product1 : Product  Inputs=3
  Product2 : Product  Inputs=3
  theta-dot-dot : Outport
  wires:
  U3,M/1 -> Product/2
  Constant/1 -> Product/1
  Omega-r/1 -> Product1/2
  Constant1/1 -> Product1/1
  Phi-dot/1 -> Product1/3
  Phi-dot1/1 -> Product2/1
  Psi-dot/1 -> Product2/2
  Constant2/1 -> Product2/3
  Product1/1 -> Add/2
  Product/1 -> Add/1
  Product2/1 -> Add/3
  Add/1 -> Divide/1
  Constant3/1 -> Divide/2
  Divide/1 -> theta-dot-dot/1

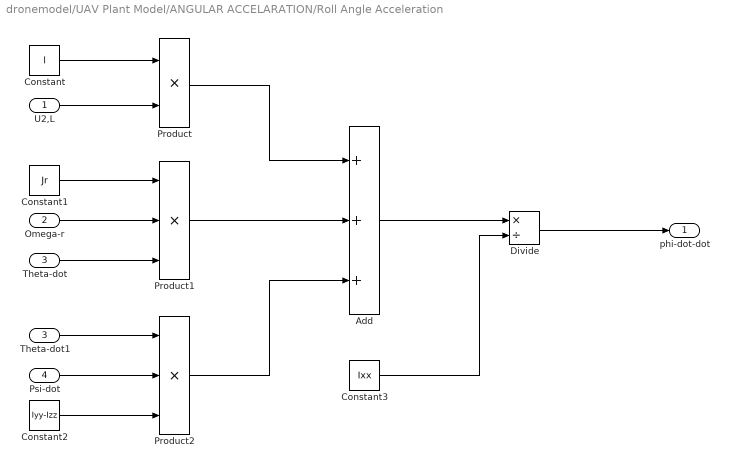
== system dronemodel/UAV Plant Model/ANGULAR ACCELARATION/Roll Angle Acceleration ==
  U2,L : Inport
  Omega-r : Inport  Port=2
  Theta-dot : Inport  Port=3
  Psi-dot : Inport  Port=4
  Add : Sum  Inputs=+++
  Constant : Constant  Value=l
  Constant1 : Constant  Value=Jr
  Constant2 : Constant  Value=Iyy-Izz
  Constant3 : Constant  Value=Ixx
  Divide : Product  Inputs=*/  RndMeth=Zero  SaturateOnIntegerOverflow=on
  Product : Product
  Product1 : Product  Inputs=3
  Product2 : Product  Inputs=3
  Theta-dot1 : InportShadow  Port=3
  phi-dot-dot : Outport
  wires:
  U2,L/1 -> Product/2
  Constant/1 -> Product/1
  Theta-dot/1 -> Product1/3
  Omega-r/1 -> Product1/2
  Constant1/1 -> Product1/1
  Theta-dot1/1 -> Product2/1
  Psi-dot/1 -> Product2/2
  Constant2/1 -> Product2/3
  Product1/1 -> Add/2
  Product/1 -> Add/1
  Product2/1 -> Add/3
  Add/1 -> Divide/1
  Constant3/1 -> Divide/2
  Divide/1 -> phi-dot-dot/1

== system dronemodel/UAV Plant Model/ANGULAR ACCELARATION/Yaw Angle Acceleration ==
  "U4, N" : Inport
  Theta-dot : Inport  Port=2
  Phi-dot : Inport  Port=3
  Add : Sum
  Constant : Constant  Value=Ixx-Iyy
  Constant1 : Constant  Value=Izz
  Divide : Product  Inputs=*/  RndMeth=Zero  SaturateOnIntegerOverflow=on
  Product : Product  Inputs=3
  psi-dot-dot : Outport
  wires:
  "U4, N"/1 -> Add/1
  Product/1 -> Add/2
  Phi-dot/1 -> Product/2
  Theta-dot/1 -> Product/1
  Constant/1 -> Product/3
  Add/1 -> Divide/1
  Constant1/1 -> Divide/2
  Divide/1 -> psi-dot-dot/1

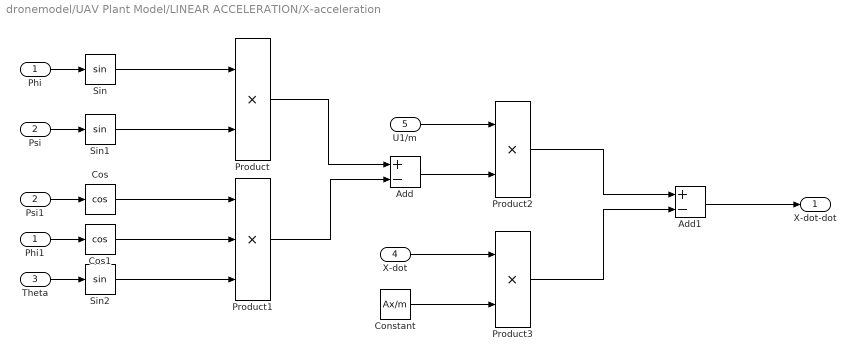
== system dronemodel/UAV Plant Model/LINEAR ACCELERATION/X-acceleration ==
  Phi : Inport
  Psi : Inport  Port=2
  Theta : Inport  Port=3
  X-dot : Inport  Port=4
  U1/m : Inport  Port=5
  Add : Sum  Inputs=+-
  Add1 : Sum  Inputs=+-
  Constant : Constant  Value=Ax/m
  Cos : Trigonometry  Operator=cos
  Cos1 : Trigonometry  Operator=cos
  Phi1 : InportShadow
  Product : Product
  Product1 : Product  Inputs=3
  Product2 : Product
  Product3 : Product
  Psi1 : InportShadow  Port=2
  Sin : Trigonometry
  Sin1 : Trigonometry
  Sin2 : Trigonometry
  X-dot-dot : Outport
  wires:
  Phi/1 -> Sin/1
  Sin/1 -> Product/1
  Psi/1 -> Sin1/1
  Sin1/1 -> Product/2
  Psi1/1 -> Cos/1
  Cos/1 -> Product1/1
  Cos1/1 -> Product1/2
  Phi1/1 -> Cos1/1
  Theta/1 -> Sin2/1
  Sin2/1 -> Product1/3
  Product/1 -> Add/1
  Product1/1 -> Add/2
  Add/1 -> Product2/2
  U1/m/1 -> Product2/1
  Constant/1 -> Product3/2
  X-dot/1 -> Product3/1
  Product3/1 -> Add1/2
  Add1/1 -> X-dot-dot/1
  Product2/1 -> Add1/1

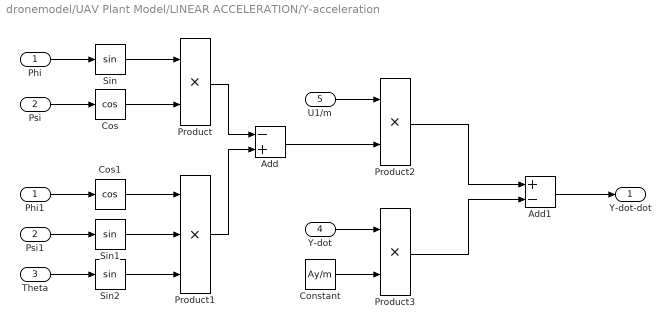
== system dronemodel/UAV Plant Model/LINEAR ACCELERATION/Y-acceleration ==
  Phi : Inport
  Psi : Inport  Port=2
  Theta : Inport  Port=3
  Y-dot : Inport  Port=4
  U1/m : Inport  Port=5
  Add : Sum  Inputs=-+
  Add1 : Sum  Inputs=+-
  Constant : Constant  Value=Ay/m
  Cos : Trigonometry  Operator=cos
  Cos1 : Trigonometry  Operator=cos
  Phi1 : InportShadow
  Product : Product
  Product1 : Product  Inputs=3
  Product2 : Product
  Product3 : Product
  Psi1 : InportShadow  Port=2
  Sin : Trigonometry
  Sin1 : Trigonometry
  Sin2 : Trigonometry
  Y-dot-dot : Outport
  wires:
  Phi/1 -> Sin/1
  Psi/1 -> Cos/1
  Sin/1 -> Product/1
  Cos/1 -> Product/2
  Phi1/1 -> Cos1/1
  Cos1/1 -> Product1/1
  Sin1/1 -> Product1/2
  Psi1/1 -> Sin1/1
  Theta/1 -> Sin2/1
  Sin2/1 -> Product1/3
  Product/1 -> Add/1
  Product1/1 -> Add/2
  Add/1 -> Product2/2
  U1/m/1 -> Product2/1
  Y-dot/1 -> Product3/1
  Constant/1 -> Product3/2
  Add1/1 -> Y-dot-dot/1
  Product2/1 -> Add1/1
  Product3/1 -> Add1/2

== system dronemodel/UAV Plant Model/LINEAR ACCELERATION/Z-acceleration ==
  Theta : Inport
  Phi : Inport  Port=2
  Z-dot : Inport  Port=3
  U1/m : Inport  Port=4
  Add : Sum  Inputs=-+
  Add1 : Sum  Inputs=+-
  Constant : Constant  Value=g
  Constant1 : Constant  Value=Az/m
  Cos : Trigonometry  Operator=cos
  Cos1 : Trigonometry  Operator=cos
  Product : Product  Inputs=3
  Product1 : Product
  Z-dot-dot : Outport
  wires:
  Theta/1 -> Cos/1
  Cos/1 -> Product/1
  Phi/1 -> Cos1/1
  Cos1/1 -> Product/2
  U1/m/1 -> Product/3
  Product/1 -> Add/2
  Constant/1 -> Add/1
  Z-dot/1 -> Product1/1
  Constant1/1 -> Product1/2
  Add/1 -> Add1/1
  Product1/1 -> Add1/2
  Add1/1 -> Z-dot-dot/1
